simulink model "FCS_MPC_6ph_CIL_FCS_reduced"  (R2022a)
settings: Solver=ode23t  StartTime=0.0  StopTime=0.1  RelTol=1e-3  AbsTol=1e-3  EnableMultiTasking=on
values from neighbouring files (symbols this model uses):
  f_c = 100000    [Params_testbench.m]
  L_d = 0.0001473    [Params_testbench.m]
  L_q = 0.0001484    [Params_testbench.m]
  L_x = 0.00005566    (= 5.566e-05)    [Params_testbench.m]
  L_y = L_x    (= 5.566e-05)    [Params_testbench.m]
  p = 5    [Params_testbench.m]
  psi_pm = 0.0048    [Params_testbench.m]
  R_ph = 0.1278    [Params_testbench.m]
  u_dc = 36.0    (= 36)    [Params_testbench.m]
libraries: nesl_utility x39, fl_lib x32, hdlsllib x20, ee_lib x12, simulink x2, spsAlphaBetaZerotodq0Lib x1
(part 1 of 3)
settings Model: Creator=Michael Hoerner  LastModifiedBy=Andre Merx
settings SolverCC: AutoScaleAbsTol=off  AlgebraicLoopSolver=TrustRegion  DecoupledContinuousIntegration=on  MinimalZcImpactIntegration=on
settings DataIOCC: LimitDataPoints=on  MaxDataPoints=10000  ReturnWorkspaceOutputs=off
settings OptimizationCC: DefaultParameterBehavior=Inlined  PassReuseOutputArgsAs=Individual arguments  OptimizeBlockOrder=speed  DifferentSizesBufferReuse=on  EfficientTunableParamExpr=on
settings DebuggingCC: ParameterTunabilityLossMsg=error  UnconnectedInputMsg=warning  UnconnectedOutputMsg=warning  UnconnectedLineMsg=warning  AllowSymbolicDim=off  SFUnexpectedBacktrackingDiag=warning  SFNoUnconditionalDefaultTransitionDiag=warning  SFExecutionAtInitializationDiag=none  SFMachineParentedDataDiag=warning  ArithmeticOperatorsInVariantConditions=warning
settings HardwareCC: ProdBitPerPointer=32  ProdBitPerSizeT=32  ProdBitPerPtrDiffT=32  ProdLargestAtomicInteger=Long  ProdLargestAtomicFloat=Double  ProdWordSize=32  ProdHWDeviceType=ARM Compatible->ARM Cortex-R
settings SFSimCC: SimUseLocalCustomCode=off  MATLABDynamicMemAlloc=off  CustomCodeUndefinedFunction=UseInterfaceOnly
settings RTWCC: SystemTargetFile=ert.tlc  GenCodeOnly=on  TemplateMakefile=ert_default_tmf  GenerateReport=on  RTWUseLocalCustomCode=off  BuildConfiguration=Faster Runs  IncludeHyperlinkInReport=on  GenerateTraceInfo=on  GenerateTraceReport=on  GenerateTraceReportSl=on  GenerateTraceReportSf=on  GenerateTraceReportEml=on  GenerateCodeMetricsReport=on  CheckMdlBeforeBuild=Warning  DLArmComputeVersion=19.05
settings CodeAppCC: ForceParamTrailComments=on  IgnoreCustomStorageClasses=off  OperatorAnnotations=on  SimulinkDataObjDesc=on  SFDataObjDesc=on  MATLABFcnDesc=on  InsertBlockDesc=on  StateflowObjectComments=on  MATLABSourceComments=on  EnableCustomComments=on  ReqsInCode=on
settings ERTTargetCC: CodeReplacementLibrary=GNU C99 extensions  GenerateSampleERTMain=on  SuppressErrorStatus=on  IncludeFileDelimiter=UseQuote  CodeInterfacePackaging=Reusable function  SupportNonFinite=off  MultiInstanceErrorCode=Warning  RootIOFormat=Part of model data structure  ERTCustomFileTemplate=example_file_process.tlc  GlobalDataDefinition=InSourceFile  GlobalDataReference=InSourceFile  ERTFilePackagingFormat=CompactWithDataFile
settings ConfigComp: CovMetricSettings=dw  CovSaveCumulativeToWorkspaceVar=on  CovSaveSingleToWorkspaceVar=on  CovExternalEMLEnable=off  CovSFcnEnable=off
settings SimscapeCC: SimscapeLogDataHistory=10000

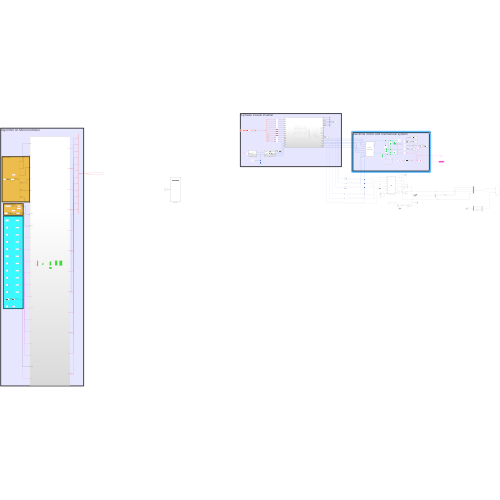
[thumbnail: Simulink's stored preview of the top-level diagram]
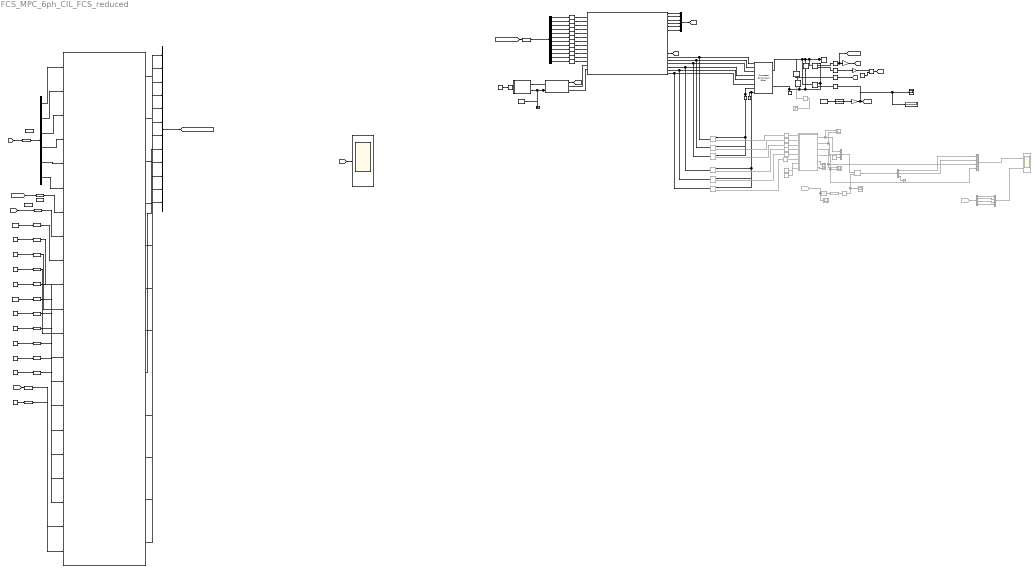
== system FCS_MPC_6ph_CIL_FCS_reduced ==
  note: electrical motor and mechanical system
  note: 6-phase 2-level inverter
  note: Von IP-Core ADC
  note: AXI
  note: Algorithm on Microcontroller
  note: Von IP-Core IncreEncoder
  6ph_Inverter : Subsystem
  6ph_PMSM_30deg_VSD1 : MATLAB Function  Commented=on  TreatAsAtomicUnit=on
  Alpha-Beta-Zero to dq0 : spsAlphaBetaZerotodq0Lib/Alpha-Beta-Zero to dq0  Commented=on  Alignment=Aligned with phase A axis
      settings: SourceProductBaseCode=PS
  Constant : Constant  Value=2*pi
  Constant10 : Constant  Commented=on  Value=1/3
  Constant11 : Constant  Value=R_ph
  Constant12 : Constant  Value=1/f_c
  Constant13 : Constant  Value=psi_pm
  Constant15 : Constant  Value=L_q
  Constant16 : Constant  Value=L_x
  Constant17 : Constant  Value=L_y
  Constant2 : Constant  Value=L_d
  Constant6 : Constant  Value=u_dc
  Constant8 : Constant  Commented=on  Value=0  OutDataTypeStr=single
  Constant9 : Constant  Commented=on
  DC_link : Subsystem
  Data Type Conversion{1..3,7,10..11,22..23,28..31,38..41} (16 alike) : DataTypeConversion  OutDataTypeStr=single  SaturateOnIntegerOverflow=off  RndMeth=Floor
  Data Type Conversion4 : DataTypeConversion  Commented=on  OutDataTypeStr=single  SaturateOnIntegerOverflow=off  RndMeth=Floor
  Data Type Conversion42 : DataTypeConversion  OutDataTypeStr=double  SaturateOnIntegerOverflow=off  RndMeth=Floor
  Data Type Conversion6 : DataTypeConversion  OutDataTypeStr=fixdt(1,24,11)  SaturateOnIntegerOverflow=off  RndMeth=Floor
  Data Type Conversion8 : DataTypeConversion  OutDataTypeStr=fixdt(1,24,20)  SaturateOnIntegerOverflow=off  RndMeth=Floor
  Data Type Conversion9 : DataTypeConversion  OutDataTypeStr=fixdt(1,18,11)  SaturateOnIntegerOverflow=off  RndMeth=Floor
  DelayValue1 : Delay  Commented=on  DelayLength=1
  Demux : Demux  Commented=on
  Demux1 : Demux  Commented=on  Outputs=3
  Demux2 : Demux  Outputs=12
  Demux6 : Demux  Outputs=6
  Display : Display
  Electrical Reference1 : fl_lib/Electrical/Electrical Elements/Electrical Reference
      settings: SourceProductBaseCode=PW,SS,VE
  From1 : From  Commented=on  GotoTag=theta_el
  From2 : From  Commented=on  GotoTag=v_opt
  Gain : Gain  Gain=30/pi
  Gain7 : Gain  Gain=p
  Gain8 : Gain  Gain=pi/30
  Ideal Angular Velocity Source1 : fl_lib/Mechanical/Mechanical Sources/Ideal Angular Velocity Source
      settings: SourceProductBaseCode=PW,SS,VE
  Ideal Rotational Motion Sensor1 : fl_lib/Mechanical/Mechanical Sensors/Ideal Rotational Motion Sensor  wrap_angle=simscape.enum.onoff.off  offset=0 deg
      settings: SourceProductBaseCode=PW,SS,VE
  Ideal Torque Sensor : fl_lib/Mechanical/Mechanical Sensors/Ideal Torque Sensor
      settings: SourceProductBaseCode=PW,SS,VE
  Ideal Torque Source : fl_lib/Mechanical/Mechanical Sources/Ideal Torque Source
      settings: SourceProductBaseCode=PW,SS,VE
  Inertia1 : fl_lib/Mechanical/Rotational Elements/Inertia  inertia=J kg*m^2  num_ports=foundation.enum.numPorts2.one  w_specify=off  w_priority=High  w=0 rad/s  w_nominal_specify=off  w_nominal_unit=rad/s  w_nominal_value=1  t_specify=off  t_priority=None  t=0 N*m  t_nominal_specify=off  t_nominal_unit=N*m  t_nominal_value=1
      settings: SourceProductBaseCode=PW,SS,VE
  Mechanical Rotational Reference1 : fl_lib/Mechanical/Rotational Elements/Mechanical Rotational Reference
      settings: SourceProductBaseCode=PW,SS,VE
  Microcontroller Software : Subsystem
  Mod : Math  Operator=mod
  Mux : Mux  Commented=on
  Mux1 : Mux  Inputs=6
  Mux2 : Mux  Commented=on
  Mux3 : Mux  Commented=on  Inputs=3
  Mux7 : Mux  Inputs=12
  Open Circuit : fl_lib/Electrical/Electrical Elements/Open Circuit  v_specify=off  v_priority=None  v=0 V  v_nominal_specify=off  v_nominal_unit=V  v_nominal_value=1
      settings: SourceProductBaseCode=PW,SS,VE
  Open Circuit1 : fl_lib/Electrical/Electrical Elements/Open Circuit  v_specify=off  v_priority=None  v=0 V  v_nominal_specify=off  v_nominal_unit=V  v_nominal_value=1
      settings: SourceProductBaseCode=PW,SS,VE
  PS-Simulink Converter{1..5,9} (6 alike) : nesl_utility/PS-Simulink Converter  Commented=on  PhysicalDomain=network_engine_domain  SubClassName=ps_output  LeftPortType=input  RightPortType=output  PseudoPeriodic=off  Frequencies=[]  VectorFormat=1-D array  Unit=V  AffineConversion=off
      settings: SourceProductBaseCode=SS,PW,VE
  PS-Simulink Converter6 : nesl_utility/PS-Simulink Converter  PhysicalDomain=network_engine_domain  SubClassName=ps_output  LeftPortType=input  RightPortType=output  PseudoPeriodic=off  Frequencies=[]  VectorFormat=1-D array  Unit=1  AffineConversion=off
      settings: SourceProductBaseCode=SS,PW,VE
  PS-Simulink Converter7 : nesl_utility/PS-Simulink Converter  PhysicalDomain=network_engine_domain  SubClassName=ps_output  LeftPortType=input  RightPortType=output  PseudoPeriodic=off  Frequencies=[]  VectorFormat=1-D array  Unit=1  AffineConversion=off
      settings: SourceProductBaseCode=SS,PW,VE
  PS-Simulink Converter8 : nesl_utility/PS-Simulink Converter  PhysicalDomain=network_engine_domain  SubClassName=ps_output  LeftPortType=input  RightPortType=output  PseudoPeriodic=off  Frequencies=[]  VectorFormat=1-D array  Unit=1  AffineConversion=off
      settings: SourceProductBaseCode=SS,PW,VE
  Power_Source : Subsystem
  Rotational Friction : fl_lib/Mechanical/Rotational Elements/Rotational Friction  brkwy_trq=0.0622476 N*m  brkwy_vel=0.1 rad/s  Col_trq=0.03460117 N*m  visc_coef=0.00026373 N*m/(rad/s)  w_specify=off  w_priority=None  w=0 rad/s  w_nominal_specify=off  w_nominal_unit=rad/s  w_nominal_value=1  t_specify=off  t_priority=None  t=0 N*m  t_nominal_specify=off  t_nominal_unit=N*m  t_nominal_value=1
      settings: SourceProductBaseCode=PW,SS,VE
  Scope : Scope
  Scope1 : Scope  Commented=on  NumInputPorts=2
  Scope2 : Scope  Commented=on  NumInputPorts=2
  Scope3 : Scope  Commented=on  NumInputPorts=2
  Scope4 : Scope  Commented=on
  Scope5 : Scope  Commented=on
  Simscape Component : SimscapeComponentBlock  SourceFile=SixPhase_PMSM  ComponentPath=SixPhase_PMSM  ComponentVariants=SixPhase_PMSM  ComponentVariantNames=SixPhase_PMSM  ClassName=SixPhase_PMSM  SchemaVersion=1  Rs=R_ph Ohm  Ld=L_d H  Lq=L_q H  Lx=L_x H  Ly=L_y H  psiPM=psi_pm Wb  np=p  theta_m_specify=off  theta_m_priority=None  theta_m=0 rad  theta_m_nominal_specify=off  theta_m_nominal_unit=rad  theta_m_nominal_value=1
      settings: CopyFcn=simscape.engine.sli.internal.componentblockcallback(gcbh,'COPY')  PreCopyFcn=simscape.engine.sli.internal.componentblockcallback(gcbh,'PRECOPY')  PreDeleteFcn=simscape.engine.sli.internal.componentblockcallback(gcbh,'PREDELETE')  InternalSimscapePortConfiguration="{\"Bottom\":[],\"Left\":[{\"id\":\"a1\",\"label\":\"a1\",\"type\":\"foundation.electrical.electrical\"},{\"id\":\"b1\",\"label\":\"b1\",\"type\":\"foundation.electrical.electrical\"},{\"id\":\"c1\",\"label\":\"c1\",\"type\":\"foundation.electrical.electrical\"},{\"id\":\"a2\",\"label\":\"a2\",\"type\":\"foundation.electrical.electrical\"},{\"id\":\"b2\",\"label\":\"b2\",\"type\":\"foundation.electrical.electrical\"},{\"id\":\"c2\",\"label\":\"c2\",\"type\":\"foundation.electrical.electrical\"},{\"id\":\"n1\",\"label\":\"n1\",\"type\":\"foundation.electrical.electrical\"},{\"id\":\"n2\",\"label\":\"n2\",\"type\":\"foundation.electrical.electrical\"}],\"Right\":[{\"id\":\"R\",\"label\":\"R\",\"type\":\"foundation.mechanical.rotational.rotational\"},{\"id\":\"C\",\"label\":\"C\",\"type\":\"foundation.mechanical.rotational.rotational\"}],\"Top\":[]}"
      mask Type: SixPhase_PMSM
  Simulink-PS Converter{,2..7,11..12,17..20} (13 alike) : nesl_utility/Simulink-PS Converter  PhysicalDomain=network_engine_domain  SubClassName=ps_input  LeftPortType=input  RightPortType=output  PseudoPeriodic=off  Frequencies=[]  NoiseDistribution=none  NoiseParameters=[]  Unit=1  AffineConversion=off  FilteringAndDerivatives=provide  SimscapeFilterOrder=1  InputFilterTimeConstant=0.001  UdotUserProvided=0
      settings: SourceProductBaseCode=SS,PW,VE
  Simulink-PS Converter1 : nesl_utility/Simulink-PS Converter  Commented=on  PhysicalDomain=network_engine_domain  SubClassName=ps_input  LeftPortType=input  RightPortType=output  PseudoPeriodic=off  Frequencies=[]  NoiseDistribution=none  NoiseParameters=[]  Unit=1  AffineConversion=off  FilteringAndDerivatives=filter  SimscapeFilterOrder=1  InputFilterTimeConstant=0.001  UdotUserProvided=0
      settings: SourceProductBaseCode=SS,PW,VE
  Simulink-PS Converter10 : nesl_utility/Simulink-PS Converter  PhysicalDomain=network_engine_domain  SubClassName=ps_input  LeftPortType=input  RightPortType=output  PseudoPeriodic=off  Frequencies=[]  NoiseDistribution=none  NoiseParameters=[]  Unit=1  AffineConversion=off  FilteringAndDerivatives=filter  SimscapeFilterOrder=1  InputFilterTimeConstant=0.001  UdotUserProvided=0
      settings: SourceProductBaseCode=SS,PW,VE
  Solver Configuration1 : nesl_utility/Solver Configuration  PhysicalDomain=network_engine_domain  SubClassName=solver  LeftPortType=input  RightPortType=generic  Tones=[]  Harmonics=[]  SimulateNoise=off  Profile=off  UseLocalSampling=off  EnableSwitchedLinearOptims=on  FrequencyDomain=off  UseCCode=off  RelTol=0.001  AbsTol=1e-06  MinStep=1e-09  ToWorkspace=off  RevertToSquareIcSolve=off  NumHomotopyIterations=100  PhasorMode=off  PhasorModeNumHarmonics=1  IndexReductionMethod=DerivativeReplacement  DoDC=off  ResidualTolerance=1e-09  UseLocalSolver=off  LocalSolverChoice=NE_BACKWARD_EULER_ADVANCER  LocalSolverSampleTime=1e-6  DoFixedCost=off  MaxNonlinIter=3  MaxModeIter=2  ComputeImpulses=off  ImpulseIterations=2  LinearAlgebra=Sparse  LinearAlgebraNumThread=0  EquationFormulation=NE_TIME_EF  DelaysMemoryBudget=1024  AutomaticFiltering=on  FilteringTimeConstant=0.001  PartitionStorageMethod=AS_NEEDED  PartitionMemoryBudget=1024  PartitionMethod=FAST
      settings: SourceProductBaseCode=SS,PW,VE
  Step1 : Step  Commented=on  Time=0.08  After=-0.5  SampleTime=0
  Terminator5 : Terminator  Commented=on
  Terminator6 : Terminator  Commented=on
  Terminator7 : Terminator  Commented=on
  Transfer Fcn : TransferFcn  Denominator=[0.0005 1]
  Unit Delay1 : UnitDelay  Commented=on  SampleTime=1/f_c  HasFrameUpgradeWarning=on
  Voltage Sensor{,1..5} (6 alike) : fl_lib/Electrical/Electrical Sensors/Voltage Sensor  Commented=on
      settings: SourceProductBaseCode=PW,SS,VE
  id_ref1 : Constant  Value=0
  iq_ref1 : Constant  Value=10
  ix_ref : Constant  Value=0
  iy_ref : Constant  Value=0
  n_ref : Constant  Value=3000
  phase_currents : Scope
  pole_pairs : Constant  Value=p
  wires:
  DC_link/1(u_dc_link_measured) -> [u_dc_link]
  Constant6/1 -> Simulink-PS Converter/1
  PS-Simulink Converter7/1 -> Gain7/1  "theta_m"
  Gain7/1 -> Mod/1  "theta_el"
  Gain8/1 -> Simulink-PS Converter10/1, Display/1, Scope/1, [omega_m]
  PS-Simulink Converter6/1 -> Gain/1, [omega_m_m]  "omega_m"
  PS-Simulink Converter8/1 -> [torque]
  [i_ph] -> phase_currents/1
  n_ref/1 -> Transfer Fcn/1
  Gain/1 -> [n_RPM]
  Step1/1 -> Simulink-PS Converter1/1
  6ph_Inverter/1(i_1) -> Mux1/1  "i_a1"
  6ph_Inverter/6(i_6) -> Mux1/6  "i_c2"
  6ph_Inverter/4(i_4) -> Mux1/4  "i_a2"
  Demux2/6 -> Simulink-PS Converter17/1
  Demux2/5 -> Simulink-PS Converter7/1
  6ph_Inverter/13(i_dc) -> [i_dc]
  Demux2/7 -> Simulink-PS Converter18/1
  6ph_Inverter/3(i_3) -> Mux1/3  "i_c1"
  6ph_Inverter/5(i_5) -> Mux1/5  "i_b2"
  Demux2/3 -> Simulink-PS Converter5/1
  [Switching_states_IP_Cores] -> Data Type Conversion42/1
  6ph_Inverter/2(i_2) -> Mux1/2  "i_b1"
  Demux2/2 -> Simulink-PS Converter4/1
  Demux2/11 -> Simulink-PS Converter11/1
  Demux2/12 -> Simulink-PS Converter12/1
  Demux2/8 -> Simulink-PS Converter19/1
  Demux2/9 -> Simulink-PS Converter20/1
  Demux2/4 -> Simulink-PS Converter6/1
  Demux2/10 -> Simulink-PS Converter3/1
  Demux2/1 -> Simulink-PS Converter2/1
  Mux1/1 -> [i_ph]
  Constant/1 -> Mod/2
  Mod/1 -> [theta_el]
  iq_ref1/1 -> Data Type Conversion30/1
  Data Type Conversion30/1 -> Microcontroller Software/17(iq_ref)
  Constant11/1 -> Data Type Conversion22/1
  Constant13/1 -> Data Type Conversion28/1
  [u_dc_link] -> Data Type Conversion7/1
  Data Type Conversion10/1 -> Microcontroller Software/10(Ld)
  Demux6/1 -> Microcontroller Software/1(i_a1)
  Data Type Conversion23/1 -> Microcontroller Software/15(SampleTime)
  Data Type Conversion22/1 -> Microcontroller Software/9(Rs)
  Constant12/1 -> Data Type Conversion23/1
  id_ref1/1 -> Data Type Conversion29/1
  Constant2/1 -> Data Type Conversion10/1
  Data Type Conversion29/1 -> Microcontroller Software/16(id_ref)
  Demux6/2 -> Microcontroller Software/2(i_b1)
  Demux6/3 -> Microcontroller Software/3(i_c1)
  Data Type Conversion28/1 -> Microcontroller Software/14(psiPM)
  Constant15/1 -> Data Type Conversion11/1
  Data Type Conversion11/1 -> Microcontroller Software/11(Lq)
  Demux6/4 -> Microcontroller Software/4(i_a2)
  Demux6/5 -> Microcontroller Software/5(i_b2)
  Demux6/6 -> Microcontroller Software/6(i_c2)
  Constant16/1 -> Data Type Conversion31/1
  Data Type Conversion31/1 -> Microcontroller Software/12(Lx)
  Constant17/1 -> Data Type Conversion38/1
  Data Type Conversion38/1 -> Microcontroller Software/13(Ly)
  pole_pairs/1 -> Data Type Conversion41/1
  Data Type Conversion39/1 -> Microcontroller Software/18(ix_ref)
  ix_ref/1 -> Data Type Conversion39/1
  Data Type Conversion40/1 -> Microcontroller Software/19(iy_ref)
  iy_ref/1 -> Data Type Conversion40/1
  Data Type Conversion41/1 -> Microcontroller Software/21(pole_pairs)
  Microcontroller Software/1(HB1T1) -> Mux7/1
  Microcontroller Software/2(HB1B1) -> Mux7/2
  Microcontroller Software/3(HB2T1) -> Mux7/3
  Microcontroller Software/4(HB2B1) -> Mux7/4
  Microcontroller Software/5(HB3T1) -> Mux7/5
  Microcontroller Software/6(HB3B1) -> Mux7/6
  Microcontroller Software/7(HB4T) -> Mux7/7
  Microcontroller Software/8(HB4B) -> Mux7/8
  Microcontroller Software/9(HB5T) -> Mux7/9
  Microcontroller Software/10(HB5B) -> Mux7/10
  Microcontroller Software/11(HB6T) -> Mux7/11
  Microcontroller Software/12(HB6B) -> Mux7/12
  Mux7/1 -> [Switching_states_IP_Cores]
  Data Type Conversion42/1 -> Demux2/1
  Constant9/1 -> 6ph_PMSM_30deg_VSD1/8(c6)
  6ph_PMSM_30deg_VSD1/6(y6) -> Terminator6/1
  6ph_PMSM_30deg_VSD1/3(y3) -> Mux/3, Scope2/1  "v_x_inverter"
  Constant10/1 -> 6ph_PMSM_30deg_VSD1/7(k6)
  6ph_PMSM_30deg_VSD1/1(y1) -> Scope3/1, Mux3/1  "i_alpha"
  6ph_PMSM_30deg_VSD1/2(y2) -> Scope3/2, Mux3/2  "i_beta"
  6ph_PMSM_30deg_VSD1/4(y4) -> Scope2/2, Mux/4  "v_y_inverter"
  Mux3/1 -> Alpha-Beta-Zero to dq0/1
  Constant8/1 -> Mux3/3
  6ph_PMSM_30deg_VSD1/5(y5) -> Terminator5/1
  Demux1/2 -> Mux/2  "v_q_inverter"
  Demux1/3 -> Terminator7/1
  Alpha-Beta-Zero to dq0/1 -> Demux1/1
  Demux1/1 -> Mux/1  "v_d_inverter"
  PS-Simulink Converter1/1 -> 6ph_PMSM_30deg_VSD1/1(u1)
  PS-Simulink Converter2/1 -> 6ph_PMSM_30deg_VSD1/2(u2)
  PS-Simulink Converter3/1 -> 6ph_PMSM_30deg_VSD1/3(u3)
  PS-Simulink Converter4/1 -> 6ph_PMSM_30deg_VSD1/4(u4)
  PS-Simulink Converter5/1 -> 6ph_PMSM_30deg_VSD1/5(u5)
  PS-Simulink Converter9/1 -> 6ph_PMSM_30deg_VSD1/6(u6)
  Unit Delay1/1 -> Data Type Conversion4/1
  Data Type Conversion4/1 -> DelayValue1/1
  Mux/1 -> Scope1/1
  From2/1 -> Demux/1
  Demux/1 -> Mux2/1  "v_d_MPC"
  Demux/2 -> Mux2/2  "v_q_MPC"
  Demux/3 -> Mux2/3  "v_x_MPC"
  Demux/4 -> Mux2/4  "v_y_MPC"
  Mux2/1 -> Scope1/2
  From1/1 -> Scope5/1, Unit Delay1/1  "End_Cycle"
  DelayValue1/1 -> Alpha-Beta-Zero to dq0/2, Scope4/1  "End_Cycle"
  [i_ph] -> Data Type Conversion1/1  "End_Cycle"
  [theta_el] -> Data Type Conversion3/1  "End_Cycle"
  [omega_m_m] -> Data Type Conversion2/1  "fc"
  Data Type Conversion7/1 -> Microcontroller Software/20(u_dc_link)
  Data Type Conversion1/1 -> Demux6/1  "fc"
  Data Type Conversion3/1 -> Microcontroller Software/8(theta_el)
  Data Type Conversion2/1 -> Microcontroller Software/7(omega_m)
  Transfer Fcn/1 -> Gain8/1
  connections:
  DC_link/LConn2 -- Power_Source/RConn2 -- Solver Configuration1/RConn1 -- Electrical Reference1/LConn1
  Inertia1/LConn1 -- Ideal Torque Sensor/LConn1 -- Simscape Component/RConn1 -- Ideal Angular Velocity Source1/LConn1 -- Rotational Friction/LConn1 -- Ideal Rotational Motion Sensor1/LConn1
  Ideal Rotational Motion Sensor1/RConn1 -- Ideal Angular Velocity Source1/RConn2 -- Rotational Friction/RConn1 -- Simscape Component/RConn2 -- Mechanical Rotational Reference1/LConn1 -- Ideal Torque Source/RConn2
  Power_Source/RConn1 -- DC_link/LConn1
  PS-Simulink Converter6/LConn1 -- Ideal Rotational Motion Sensor1/RConn2
  Simulink-PS Converter/RConn1 -- Power_Source/LConn1
  6ph_Inverter/LConn13 -- DC_link/RConn1
  6ph_Inverter/LConn14 -- DC_link/RConn2
  PS-Simulink Converter7/LConn1 -- Ideal Rotational Motion Sensor1/RConn3
  Simulink-PS Converter10/RConn1 -- Ideal Angular Velocity Source1/RConn1
  PS-Simulink Converter8/LConn1 -- Ideal Torque Sensor/RConn2
  Simulink-PS Converter1/RConn1 -- Ideal Torque Source/RConn1
  Ideal Torque Source/LConn1 -- Ideal Torque Sensor/RConn1
  Simscape Component/LConn8 -- Voltage Sensor5/RConn2 -- Voltage Sensor4/RConn2 -- Voltage Sensor3/RConn2 -- Open Circuit1/LConn1
  6ph_Inverter/RConn2 -- Voltage Sensor1/LConn1 -- Simscape Component/LConn2
  Simscape Component/LConn7 -- Voltage Sensor2/RConn2 -- Voltage Sensor1/RConn2 -- Voltage Sensor/RConn2 -- Open Circuit/LConn1
  6ph_Inverter/RConn1 -- Simscape Component/LConn1 -- Voltage Sensor/LConn1
  6ph_Inverter/RConn4 -- Voltage Sensor3/LConn1 -- Simscape Component/LConn4
  6ph_Inverter/RConn5 -- Voltage Sensor4/LConn1 -- Simscape Component/LConn5
  Simulink-PS Converter7/RConn1 -- 6ph_Inverter/LConn5
  Simulink-PS Converter12/RConn1 -- 6ph_Inverter/LConn12
  Simulink-PS Converter20/RConn1 -- 6ph_Inverter/LConn9
  Simulink-PS Converter17/RConn1 -- 6ph_Inverter/LConn6
  Simulink-PS Converter11/RConn1 -- 6ph_Inverter/LConn11
  Simulink-PS Converter19/RConn1 -- 6ph_Inverter/LConn8
  Simulink-PS Converter6/RConn1 -- 6ph_Inverter/LConn4
  Simulink-PS Converter3/RConn1 -- 6ph_Inverter/LConn10
  Simulink-PS Converter4/RConn1 -- 6ph_Inverter/LConn2
  Simscape Component/LConn3 -- 6ph_Inverter/RConn3 -- Voltage Sensor2/LConn1
  Simscape Component/LConn6 -- Voltage Sensor5/LConn1 -- 6ph_Inverter/RConn6
  Simulink-PS Converter5/RConn1 -- 6ph_Inverter/LConn3
  Simulink-PS Converter2/RConn1 -- 6ph_Inverter/LConn1
  Simulink-PS Converter18/RConn1 -- 6ph_Inverter/LConn7
  Voltage Sensor/RConn1 -- PS-Simulink Converter1/LConn1
  Voltage Sensor1/RConn1 -- PS-Simulink Converter2/LConn1
  Voltage Sensor2/RConn1 -- PS-Simulink Converter3/LConn1
  Voltage Sensor3/RConn1 -- PS-Simulink Converter4/LConn1
  Voltage Sensor4/RConn1 -- PS-Simulink Converter5/LConn1
  Voltage Sensor5/RConn1 -- PS-Simulink Converter9/LConn1

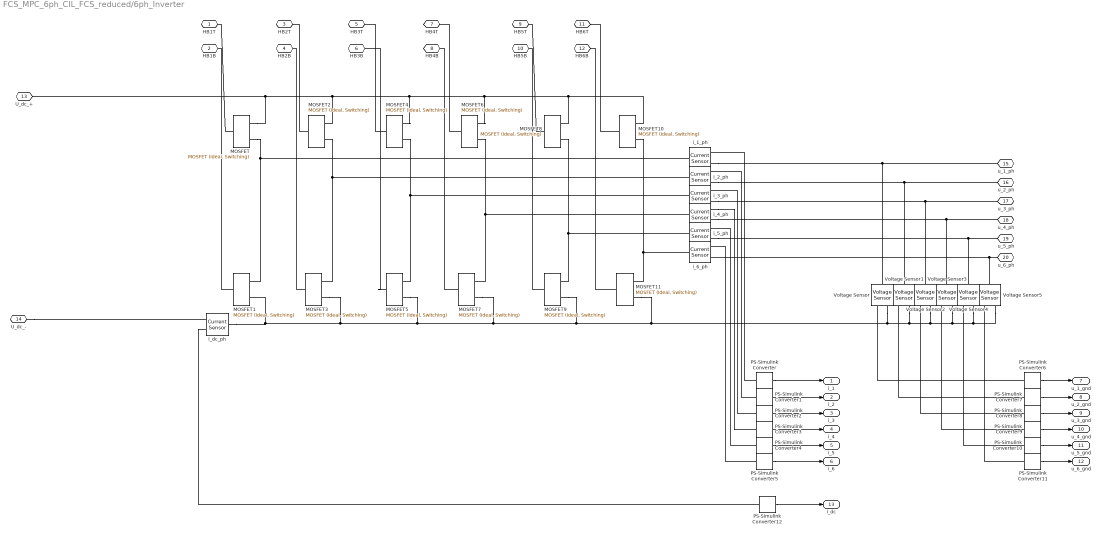
== system FCS_MPC_6ph_CIL_FCS_reduced/6ph_Inverter ==
  MOSFET{,1..11} (12 alike) : ee_lib/Semiconductors & Converters/MOSFET (Ideal, Switching)  Rds=RDSon Ohm  Goff=1e-6 1/Ohm  Vth=0.7 V  diode_param=1  diode_Vf=0.8 V  diode_Ron=0.001 Ohm  diode_Goff=1e-5 1/Ohm  diode_C=5e-8 F  diode_iRM=-235 A  diode_iF=300 A  diode_idot=-50 A/us  diode_trr_param=1  diode_trr_factor=3  diode_trr=15 us  diode_Qrr=1.5e+3 s*uA  thermal_loss_option=ee.enum.converters.thermalLossOption.constantvalues  Von_data=[0, 1.1, 1.3, 1.45, 1.75, 2.25, 2.7; 0, 1, 1.15, 1.35, 1.7, 2.35, 3] V  Tj=[298.15, 398.15] K  Iout_data=[0, 10, 50, 100, 200, 400, 600] A  Eon_data=[0, .29, 1.43, 2.86, 5.71, 13.14, 22.86; 0, .57, 2.63, 5.14, 10.29, 20.57, 30.29] * 1e-3 J  Eoff_data=[0, .21, 1.07, 2.14, 4.29, 9.86, 17.14; 0, .43, 1.97, 3.86, 7.71, 15.43, 22.71] * 1e-3 J  Tj_loss=[298.15, 398.15] K  Iout_data_loss=[0, 10, 50, 100, 200, 400, 600] A  Eon_scalar=22.86e-3 J  Eoff_scalar=17.14e-3 J  Voff=300 V  Iout_scalar=600 A  diodeModelType=ee.enum.converters.diodeModelType.pwl  diodeTableType=ee.enum.diode.tableType.IfMat  diode_IfMat=[.07, .12, .19, 1.75, 4.24, 7.32, 11.2; .16, .3, .72, 2.14, 4.02, 6.35, 9.12] A  diode_VfMat=[.9, 1.15, 1.25, 1.5, 1.75, 2.17, 2.6, 2.85; .58, .68, .75, 1.1, 1.38, 1.77, 2.27, 2.7] V  diode_TjVec=[25, 125] degC  diode_VfVec=[.5, .7, .9, 1.3, 1.7, 2.1, 2.5] V  diode_IfVec=[.1, .2, .5, 1, 2, 4, 7, 10] A  diode_Vr=-600 V  diode_Ls=150 nH  diode_Erec=0.03 J  thermal_network_parameterization=ee.enum.thermalNetworkTopology.external  Rth=[.03, .2] K/W  Rth_Cauer=[.03, .1, .2] K/W  Rth_Foster=[.03, .2] K/W  thermal_mass_parameterization=ee.enum.thermalNetwork.timeconstant  thermal_mass=[3, 25] J/K  thermal_mass_Cauer=[3, 10, 25] J/K  thermal_mass_Foster=[33, 50] J/K  thermal_time_constant=[.1, 5] s  thermal_time_constant_Cauer=[.1, 1, 5] s  thermal_time_constant_Foster=[1, 10] s  thermal_mass_initial_temperatures=[25, 25] degC  thermal_mass_initial_temperatures_Cauer=[25, 25, 25] degC  junction_thermal_mass=0.1 J/K  steadyState_Foster=simscape.enum.onoff.on  Tvec_initial_Foster=[25, 25, 25, 25] degC  no_thermal_network=0  junction_temperature_specify=off  junction_temperature_priority=None  junction_temperature=25 degC  junction_temperature_nominal_specify=off  junction_temperature_nominal_unit=degC  junction_temperature_nominal_value=1  vT_specify=off  vT_priority=None  vT=0 V  vT_nominal_specify=off  vT_nominal_unit=V  vT_nominal_value=1  Qj_specify=off  Qj_priority=None  Qj=0 W  Qj_nominal_specify=off  Qj_nominal_unit=W  Qj_nominal_value=1
  PS-Simulink Converter{,1..5,12} (7 alike) : nesl_utility/PS-Simulink Converter  PhysicalDomain=network_engine_domain  SubClassName=ps_output  LeftPortType=input  RightPortType=output  PseudoPeriodic=off  Frequencies=[]  VectorFormat=1-D array  Unit=A  AffineConversion=off
      settings: SourceProductBaseCode=SS,PW,VE
  PS-Simulink Converter{6..11} (6 alike) : nesl_utility/PS-Simulink Converter  PhysicalDomain=network_engine_domain  SubClassName=ps_output  LeftPortType=input  RightPortType=output  PseudoPeriodic=off  Frequencies=[]  VectorFormat=1-D array  Unit=V  AffineConversion=off
      settings: SourceProductBaseCode=SS,PW,VE
  Voltage Sensor{,1..5} (6 alike) : fl_lib/Electrical/Electrical Sensors/Voltage Sensor
      settings: SourceProductBaseCode=PW,SS,VE
  i_1_ph : fl_lib/Electrical/Electrical Sensors/Current Sensor
      settings: SourceProductBaseCode=PW,SS,VE
  i_2_ph : fl_lib/Electrical/Electrical Sensors/Current Sensor
      settings: SourceProductBaseCode=PW,SS,VE
  i_3_ph : fl_lib/Electrical/Electrical Sensors/Current Sensor
      settings: SourceProductBaseCode=PW,SS,VE
  i_4_ph : fl_lib/Electrical/Electrical Sensors/Current Sensor
      settings: SourceProductBaseCode=PW,SS,VE
  i_5_ph : fl_lib/Electrical/Electrical Sensors/Current Sensor
      settings: SourceProductBaseCode=PW,SS,VE
  i_6_ph : fl_lib/Electrical/Electrical Sensors/Current Sensor
      settings: SourceProductBaseCode=PW,SS,VE
  i_dc_ph : fl_lib/Electrical/Electrical Sensors/Current Sensor
      settings: SourceProductBaseCode=PW,SS,VE
  HB1T : PMIOPort  Side=Left
  HB1B : PMIOPort  Port=2  Side=Left
  HB2T : PMIOPort  Port=3  Side=Left
  HB2B : PMIOPort  Port=4  Side=Left
  HB3T : PMIOPort  Port=5  Side=Left
  HB3B : PMIOPort  Port=6  Side=Left
  HB4T : PMIOPort  Port=7  Side=Left
  HB4B : PMIOPort  Port=8  Side=Left
  HB5T : PMIOPort  Port=9  Side=Left
  HB5B : PMIOPort  Port=10  Side=Left
  HB6T : PMIOPort  Port=11  Side=Left
  HB6B : PMIOPort  Port=12  Side=Left
  U_dc_+ : PMIOPort  Port=13  Side=Left
  U_dc_- : PMIOPort  Port=14  Side=Left
  u_1_ph : PMIOPort  Port=15  Side=Right
  u_2_ph : PMIOPort  Port=16  Side=Right
  u_3_ph : PMIOPort  Port=17  Side=Right
  u_4_ph : PMIOPort  Port=18  Side=Right
  u_5_ph : PMIOPort  Port=19  Side=Right
  u_6_ph : PMIOPort  Port=20  Side=Right
  i_1 : Outport  VectorParamsAs1DForOutWhenUnconnected=off
  i_2 : Outport  Port=2  VectorParamsAs1DForOutWhenUnconnected=off
  i_3 : Outport  Port=3  VectorParamsAs1DForOutWhenUnconnected=off
  i_4 : Outport  Port=4  VectorParamsAs1DForOutWhenUnconnected=off
  i_5 : Outport  Port=5  VectorParamsAs1DForOutWhenUnconnected=off
  i_6 : Outport  Port=6  VectorParamsAs1DForOutWhenUnconnected=off
  u_1_gnd : Outport  Port=7  VectorParamsAs1DForOutWhenUnconnected=off
  u_2_gnd : Outport  Port=8  VectorParamsAs1DForOutWhenUnconnected=off
  u_3_gnd : Outport  Port=9  VectorParamsAs1DForOutWhenUnconnected=off
  u_4_gnd : Outport  Port=10  VectorParamsAs1DForOutWhenUnconnected=off
  u_5_gnd : Outport  Port=11  VectorParamsAs1DForOutWhenUnconnected=off
  u_6_gnd : Outport  Port=12  VectorParamsAs1DForOutWhenUnconnected=off
  i_dc : Outport  Port=13  VectorParamsAs1DForOutWhenUnconnected=off
  wires:
  PS-Simulink Converter/1 -> i_1/1
  PS-Simulink Converter1/1 -> i_2/1
  PS-Simulink Converter2/1 -> i_3/1
  PS-Simulink Converter3/1 -> i_4/1
  PS-Simulink Converter4/1 -> i_5/1
  PS-Simulink Converter5/1 -> i_6/1
  PS-Simulink Converter9/1 -> u_4_gnd/1
  PS-Simulink Converter8/1 -> u_3_gnd/1
  PS-Simulink Converter7/1 -> u_2_gnd/1
  PS-Simulink Converter6/1 -> u_1_gnd/1
  PS-Simulink Converter10/1 -> u_5_gnd/1
  PS-Simulink Converter11/1 -> u_6_gnd/1
  PS-Simulink Converter12/1 -> i_dc/1
  connections:
  MOSFET6/RConn2 -- i_4_ph/LConn1 -- MOSFET7/RConn1
  MOSFET2/RConn2 -- i_2_ph/LConn1 -- MOSFET3/RConn1
  MOSFET4/RConn2 -- i_3_ph/LConn1 -- MOSFET5/RConn1
  MOSFET5/RConn2 -- Voltage Sensor5/RConn2 -- Voltage Sensor4/RConn2 -- Voltage Sensor3/RConn2 -- Voltage Sensor2/RConn2 -- Voltage Sensor1/RConn2 -- Voltage Sensor/RConn2 -- MOSFET11/RConn2 -- MOSFET9/RConn2 -- MOSFET7/RConn2 -- i_dc_ph/LConn1 -- MOSFET1/RConn2 -- MOSFET3/RConn2
  MOSFET/RConn2 -- i_1_ph/LConn1 -- MOSFET1/RConn1
  MOSFET11/LConn1 -- HB6B/RConn1
  MOSFET8/RConn2 -- i_5_ph/LConn1 -- MOSFET9/RConn1
  MOSFET2/LConn1 -- HB2T/RConn1
  MOSFET10/RConn2 -- i_6_ph/LConn1 -- MOSFET11/RConn1
  MOSFET/LConn1 -- HB1T/RConn1
  MOSFET9/LConn1 -- HB5B/RConn1
  MOSFET5/LConn1 -- HB3B/RConn1
  MOSFET1/LConn1 -- HB1B/RConn1
  MOSFET7/LConn1 -- HB4B/RConn1
  MOSFET8/LConn1 -- HB5T/RConn1
  MOSFET4/LConn1 -- HB3T/RConn1
  MOSFET10/LConn1 -- HB6T/RConn1
  MOSFET6/LConn1 -- HB4T/RConn1
  MOSFET3/LConn1 -- HB2B/RConn1
  i_1_ph/RConn2 -- Voltage Sensor/LConn1 -- u_1_ph/RConn1
  i_2_ph/RConn2 -- u_2_ph/RConn1 -- Voltage Sensor1/LConn1
  i_3_ph/RConn2 -- u_3_ph/RConn1 -- Voltage Sensor2/LConn1
  i_4_ph/RConn2 -- Voltage Sensor3/LConn1 -- u_4_ph/RConn1
  i_5_ph/RConn2 -- Voltage Sensor4/LConn1 -- u_5_ph/RConn1
  u_6_ph/RConn1 -- i_6_ph/RConn2 -- Voltage Sensor5/LConn1
  PS-Simulink Converter/LConn1 -- i_1_ph/RConn1
  PS-Simulink Converter1/LConn1 -- i_2_ph/RConn1
  PS-Simulink Converter2/LConn1 -- i_3_ph/RConn1
  i_4_ph/RConn1 -- PS-Simulink Converter3/LConn1
  PS-Simulink Converter4/LConn1 -- i_5_ph/RConn1
  PS-Simulink Converter5/LConn1 -- i_6_ph/RConn1
  PS-Simulink Converter6/LConn1 -- Voltage Sensor/RConn1
  PS-Simulink Converter7/LConn1 -- Voltage Sensor1/RConn1
  PS-Simulink Converter8/LConn1 -- Voltage Sensor2/RConn1
  PS-Simulink Converter9/LConn1 -- Voltage Sensor3/RConn1
  PS-Simulink Converter10/LConn1 -- Voltage Sensor4/RConn1
  PS-Simulink Converter11/LConn1 -- Voltage Sensor5/RConn1
  U_dc_-/RConn1 -- i_dc_ph/RConn2
  PS-Simulink Converter12/LConn1 -- i_dc_ph/RConn1
  MOSFET6/RConn1 -- MOSFET/RConn1 -- U_dc_+/RConn1 -- MOSFET2/RConn1 -- MOSFET4/RConn1 -- MOSFET10/RConn1 -- MOSFET8/RConn1

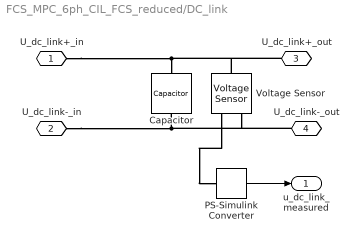
== system FCS_MPC_6ph_CIL_FCS_reduced/DC_link ==
  Capacitor : fl_lib/Electrical/Electrical Elements/Capacitor  c=C_dc_link uF  r=1e-6 Ohm  g=0 1/Ohm  i_specify=off  i_priority=None  i=0 A  i_nominal_specify=off  i_nominal_unit=A  i_nominal_value=1  v_specify=off  v_priority=None  v=0 V  v_nominal_specify=off  v_nominal_unit=V  v_nominal_value=1  vc_specify=off  vc_priority=High  vc=0 V  vc_nominal_specify=off  vc_nominal_unit=V  vc_nominal_value=1
      settings: SourceProductBaseCode=PW,SS,VE
  PS-Simulink Converter : nesl_utility/PS-Simulink Converter  PhysicalDomain=network_engine_domain  SubClassName=ps_output  LeftPortType=input  RightPortType=output  PseudoPeriodic=off  Frequencies=[]  VectorFormat=1-D array  Unit=1  AffineConversion=off
      settings: SourceProductBaseCode=SS,PW,VE
  Voltage Sensor : fl_lib/Electrical/Electrical Sensors/Voltage Sensor
      settings: SourceProductBaseCode=PW,SS,VE
  U_dc_link+_in : PMIOPort  Side=Left
  U_dc_link-_in : PMIOPort  Port=2  Side=Left
  U_dc_link+_out : PMIOPort  Port=3  Side=Right
  U_dc_link-_out : PMIOPort  Port=4  Side=Right
  u_dc_link_measured : Outport  VectorParamsAs1DForOutWhenUnconnected=off
  wires:
  PS-Simulink Converter/1 -> u_dc_link_measured/1
  connections:
  U_dc_link+_in/RConn1 -- Voltage Sensor/LConn1 -- U_dc_link+_out/RConn1 -- Capacitor/LConn1
  U_dc_link-_in/RConn1 -- Voltage Sensor/RConn2 -- U_dc_link-_out/RConn1 -- Capacitor/RConn1
  Voltage Sensor/RConn1 -- PS-Simulink Converter/LConn1

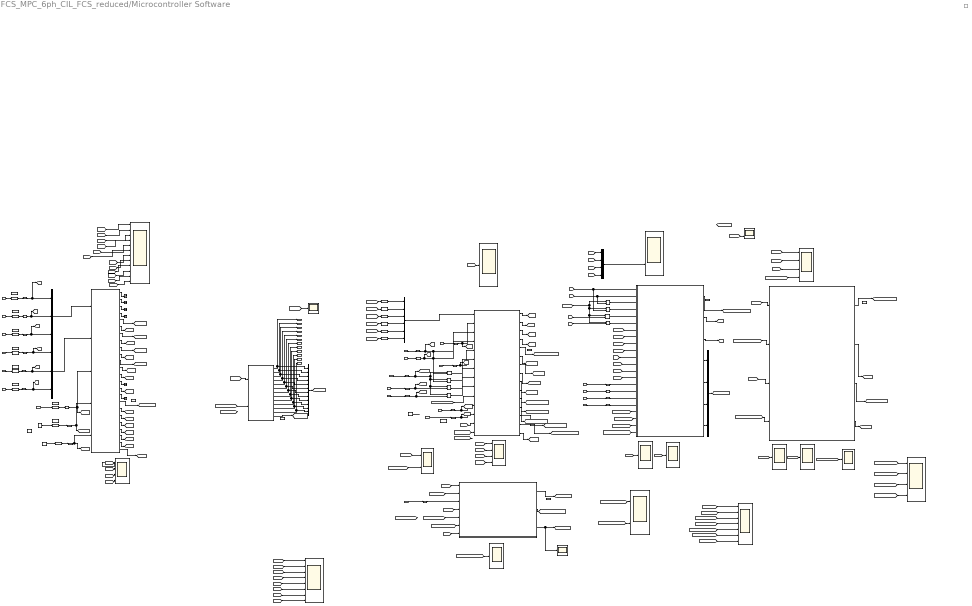
== system FCS_MPC_6ph_CIL_FCS_reduced/Microcontroller Software ==
  i_a1 : Inport
  i_b1 : Inport  Port=2
  i_c1 : Inport  Port=3
  i_a2 : Inport  Port=4
  i_b2 : Inport  Port=5
  i_c2 : Inport  Port=6
  omega_m : Inport  Port=7
  theta_el : Inport  Port=8
  Rs : Inport  Port=9
  Ld : Inport  Port=10
  Lq : Inport  Port=11
  Lx : Inport  Port=12
  Ly : Inport  Port=13
  psiPM : Inport  Port=14
  SampleTime : Inport  Port=15
  id_ref : Inport  Port=16
  iq_ref : Inport  Port=17
  ix_ref : Inport  Port=18
  iy_ref : Inport  Port=19
  u_dc_link : Inport  Port=20
  pole_pairs : Inport  Port=21
  Ablauf : Scope  NumInputPorts=7
  Constant : Constant  Value=314  OutDataTypeStr=single  SampleTime=-1
  Constant1 : Constant  Value=0  OutDataTypeStr=single  SampleTime=1/100000000
  Constant2 : Constant  Value=0  OutDataTypeStr=fixdt(1,24,20)  SampleTime=-1
  Data Type Conversion1 : DataTypeConversion  OutDataTypeStr=fixdt(1,24,11)  SaturateOnIntegerOverflow=off  RndMeth=Floor
  Data Type Conversion10 : DataTypeConversion  OutDataTypeStr=fixdt(1,18,14)  SaturateOnIntegerOverflow=off  RndMeth=Floor
  Data Type Conversion11 : DataTypeConversion  OutDataTypeStr=fixdt(1,18,14)  SaturateOnIntegerOverflow=off  RndMeth=Floor
  Data Type Conversion12 : DataTypeConversion  OutDataTypeStr=fixdt(1,24,20)  SaturateOnIntegerOverflow=off  RndMeth=Floor
  Data Type Conversion{13..18} (6 alike) : DataTypeConversion  OutDataTypeStr=fixdt(1,18,11)  SaturateOnIntegerOverflow=off  RndMeth=Floor
  Data Type Conversion{2..3,5..7,9,19..24} (12 alike) : DataTypeConversion  OutDataTypeStr=fixdt(1,27,18)  SaturateOnIntegerOverflow=off  RndMeth=Floor
  Data Type Conversion4 : DataTypeConversion  OutDataTypeStr=boolean  RndMeth=Simplest  SaturateOnIntegerOverflow=off
  Data Type Conversion8 : DataTypeConversion  OutDataTypeStr=fixdt(1,24,20)  SaturateOnIntegerOverflow=off  RndMeth=Floor
  Delay1 : Delay  DelayLength=36
  Delay2 : Delay  DelayLength=21
  Delay22 : Delay  DelayLength=3
  Delay3 : Delay  DelayLength=66
  Delay4 : Delay  DelayLength=3
  Delay6 : Delay
  Delay_compensation : Subsystem  TreatAsAtomicUnit=on
  Delay_compensation_phase_currents : Scope  NumInputPorts=4
  Divide{,1..7} (8 alike) : Product  Inputs=*/  RndMeth=Zero  SaturateOnIntegerOverflow=on
  Index : Scope
  J : Scope
  J_min_Socpe : Scope  NumInputPorts=2
  Last_applied_phase_voltages : Scope
  Last_optimal_voltages : Scope  NumInputPorts=4
  Min_cost_funcion_vergleich : Scope  NumInputPorts=4
  Min_cost_function_and_vopt2 : Subsystem  TreatAsAtomicUnit=on
  Mux : Mux  Inputs=3
  Mux1 : Mux  Inputs=3
  Mux2 : Mux
  Mux3 : Mux
  Mux4 : Mux  Inputs=12
  Mux5 : Mux  Inputs=6
  Omega_el : Scope
  Phase_voltages_per_switching_state2 : Subsystem  TreatAsAtomicUnit=on
  Phase_voltages_per_switching_states : Scope
  Prediction_and_cost_function : Subsystem  TreatAsAtomicUnit=on
  Pulse Generator3 : DiscretePulseGenerator  PulseType=Time based  Period=1/f_c  PulseWidth=0.1
  Pulse Generator4 : DiscretePulseGenerator  Commented=on  PulseType=Time based  Period=1/100000  PulseWidth=5
  Rate Transition{1..23} (23 alike) : RateTransition  OutPortSampleTime=1.0000e-08
  Switching_states : Subsystem  TreatAsAtomicUnit=on
  Terminator{,1,6..7,9..10} (6 alike) : Terminator
  VSD_and_Park_transformed_phase_currents : Scope  NumInputPorts=4
  min_Index_AXI : Scope
  min_J_AXI : Scope
  phase_currents : Scope  NumInputPorts=8
  phase_currents1 : Scope  NumInputPorts=12
  phase_currents3 : Scope  NumInputPorts=2
  phase_currents_in_delay_compensation : Scope  NumInputPorts=2
  switching_state : Scope
  theta : Scope
  theta_test : Scope  NumInputPorts=2
  vsd_and_park_tra : Subsystem  TreatAsAtomicUnit=on
  HB1T1 : Outport
  HB1B1 : Outport  Port=2
  HB2T1 : Outport  Port=3
  HB2B1 : Outport  Port=4
  HB3T1 : Outport  Port=5
  HB3B1 : Outport  Port=6
  HB4T : Outport  Port=7
  HB4B : Outport  Port=8
  HB5T : Outport  Port=9
  HB5B : Outport  Port=10
  HB6T : Outport  Port=11
  HB6B : Outport  Port=12
  wires:
  Pulse Generator3/1 -> Data Type Conversion4/1
  vsd_and_park_tra/4(i_beta_axi) -> Terminator1/1
  vsd_and_park_tra/10(i_x_axi) -> [i_x_AXI]
  vsd_and_park_tra/16(i_0_minus_axi) -> Terminator7/1
  Constant1/1 -> Data Type Conversion10/1  "i_a1_IP_Core"
  vsd_and_park_tra/12(i_y_axi) -> [i_y_AXI]
  vsd_and_park_tra/14(i_0_plus_axi) -> Terminator6/1
  vsd_and_park_tra/8(i_q_axi) -> [i_q_AXI]
  vsd_and_park_tra/6(i_d_axi) -> [i_d_AXI]
  vsd_and_park_tra/2(i_alpha_axi) -> Terminator/1
  i_a1/1 -> Data Type Conversion7/1  "i_a1_IP_Core"
  i_c2/1 -> Data Type Conversion9/1  "i_c2_IP_Core"
  i_b2/1 -> Data Type Conversion6/1  "i_b2_IP_Core"
  i_a2/1 -> Data Type Conversion5/1  "i_a2_IP_Core"
  i_c1/1 -> Data Type Conversion3/1  "i_c1_IP_Core"
  i_b1/1 -> Data Type Conversion2/1  "i_b1_IP_Core"
  vsd_and_park_tra/1(i_alpha) -> Terminator9/1  "i_alpha"
  vsd_and_park_tra/3(i_beta) -> Terminator10/1  "i_beta"
  vsd_and_park_tra/13(i_0_plus) -> [i_0_plus]  "i_0_plus"
  vsd_and_park_tra/15(i_0_minus) -> [i_0_minus]  "i_0_minus"
  vsd_and_park_tra/18(i_a1_axi) -> [i_a1_AXI]
  vsd_and_park_tra/19(i_b1_axi) -> [i_b1_AXI]
  vsd_and_park_tra/20(i_c1_axi) -> [i_c1_AXI]
  vsd_and_park_tra/21(i_a2_axi) -> [i_a2_AXI]
  vsd_and_park_tra/22(i_b2_axi) -> [i_b2_AXI]
  vsd_and_park_tra/23(i_c2_axi) -> [i_c2_AXI]
  [i_a1_AXI] -> phase_currents1/1
  [i_b1_AXI] -> phase_currents1/2
  [i_c1_AXI] -> phase_currents1/3
  [i_a2_AXI] -> phase_currents1/4
  [i_b2_AXI] -> phase_currents1/5
  [i_c2_AXI] -> phase_currents1/6
  [i_d_AXI] -> VSD_and_Park_transformed_phase_currents/1
  [i_q_AXI] -> VSD_and_Park_transformed_phase_currents/2
  [i_y_AXI] -> VSD_and_Park_transformed_phase_currents/4
  [i_x_AXI] -> VSD_and_Park_transformed_phase_currents/3
  Divide1/1 -> Delay_compensation/7(SampleTime_div_Lq_AXI)
  Divide/1 -> Delay_compensation/6(SampleTime_div_Ld_AXI)
  Delay_compensation/2(iq_k_1) -> [iq_k_1]
  Divide2/1 -> Delay_compensation/8(SampleTime_div_Lx_AXI)
  Delay_compensation/1(id_k_1) -> [id_k_1]
  Delay_compensation/4(iy_k_1) -> [iy_k_1]
  Delay_compensation/3(ix_k_1) -> [ix_k_1]
  Divide3/1 -> Delay_compensation/9(SampleTime_div_Ly_AXI)
  psiPM/1 -> Rate Transition9/1  "i_d"
  Lq/1 -> Rate Transition10/1  "i_a1_IP_Core"
  Ld/1 -> Rate Transition11/1  "i_a1_IP_Core"
  Rs/1 -> Rate Transition12/1  "i_a1_IP_Core"
  Lx/1 -> Rate Transition14/1  "i_a1_IP_Core"
  Ly/1 -> Rate Transition15/1  "i_a1_IP_Core"
  pole_pairs/1 -> Rate Transition16/1  "i_a1_IP_Core"
  Constant/1 -> ?  "i_d"
  [valid_in_ADC] -> Delay_compensation/13(valid_in_ADC)
  vsd_and_park_tra/5(i_d) -> [i_d_measured]  "i_d"
  vsd_and_park_tra/7(i_q) -> [i_q_measured]  "i_q"
  vsd_and_park_tra/9(i_x) -> [i_x_measured]  "i_x"
  vsd_and_park_tra/11(i_y) -> [i_y_measured]  "i_y"
  Delay_compensation/6(id_k_1_AXI) -> [id_k_1_AXI]
  Delay_compensation/7(iq_k_1_AXI) -> [iq_k_1_AXI]
  Delay_compensation/8(ix_k_1_AXI) -> [ix_k_1_AXI]
  Delay_compensation/9(iy_k_1_AXI) -> [iy_k_1_AXI]
  [id_k_1_AXI] -> Delay_compensation_phase_currents/1
  [iq_k_1_AXI] -> Delay_compensation_phase_currents/2
  [ix_k_1_AXI] -> Delay_compensation_phase_currents/3
  [iy_k_1_AXI] -> Delay_compensation_phase_currents/4
  [theta_el] -> Phase_voltages_per_switching_state2/1(theta_el)
  [theta_el_offset_AXI] -> Phase_voltages_per_switching_state2/2(theta_el_offset_AXI)
  u_dc_link/1 -> Rate Transition22/1  "i_a1_IP_Core"
  [done_switching_states] -> Phase_voltages_per_switching_state2/5(valid_in_delay_compensation)
  [valid_in_ADC] -> Phase_voltages_per_switching_state2/7(valid_in_ADC)
  Phase_voltages_per_switching_state2/2(phase_voltages_per_switching_state) -> [phase_voltages_per_switching_states]
  [phase_voltages_per_switching_states] -> Phase_voltages_per_switching_states/1
  Divide6/1 -> Prediction_and_cost_function/5(SampleTime_div_Lx_AXI)
  [psiPM] -> Prediction_and_cost_function/14(psiPM_AXI)
  Divide7/1 -> Prediction_and_cost_function/6(SampleTime_div_Ly_AXI)
  [Ld] -> Divide4/2, Prediction_and_cost_function/2(Ld_AXI)
  [omega_m] -> Prediction_and_cost_function/12(omega_m_measured)
  [SampleTime] -> Divide5/1, Divide7/1, Divide6/1, Divide4/1
  [Lq] -> Divide5/2, Prediction_and_cost_function/1(Lq_AXI)
  Divide4/1 -> Prediction_and_cost_function/3(SampleTime_div_Ld_AXI)
  [Rs] -> Prediction_and_cost_function/11(Rs_AXI)
  [Ly] -> Divide7/2
  [Lx] -> Divide6/2
  Prediction_and_cost_function/2(Index) -> [Index]
  Divide5/1 -> Prediction_and_cost_function/4(SampleTime_div_Lq_AXI)
  [pole_pairs] -> Prediction_and_cost_function/13(pole_pairs_AXI)
  Prediction_and_cost_function/3(J) -> [J]
  [J] -> J/1
  [Index] -> Index/1
  [id_k_1] -> Prediction_and_cost_function/7(id_k_1)
  [iq_k_1] -> Prediction_and_cost_function/8(iq_k_1)
  [ix_k_1] -> Prediction_and_cost_function/9(ix_k_1)
  [iy_k_1] -> Prediction_and_cost_function/10(iy_k_1)
  id_ref/1 -> Rate Transition18/1  "i_a1_IP_Core"
  iq_ref/1 -> Rate Transition19/1  "i_a1_IP_Core"
  ix_ref/1 -> Rate Transition20/1  "i_a1_IP_Core"
  iy_ref/1 -> Rate Transition21/1  "i_a1_IP_Core"
  [valid_in_phase_voltages] -> Prediction_and_cost_function/19(valid_in)
  [done_VSD_and_Park] -> Prediction_and_cost_function/20(Reset)
  [valid_in_ADC] -> Prediction_and_cost_function/21(valid_in_ADC)
  [phase_voltages_per_switching_states] -> Prediction_and_cost_function/22(dqxy_phase_voltage_per_switching_state)
  Min_cost_function_and_vopt2/4(Index_AXI) -> [min_Index_AXI]
  Min_cost_function_and_vopt2/2(Index) -> [min_Index]
  Min_cost_function_and_vopt2/3(voltages) -> [last_applied_optimal_voltages]
  [Index] -> Min_cost_function_and_vopt2/1(Index_in)
  [Index] -> Phase_voltages_per_switching_state2/4(Index)
  [valid_in_prediction_and_cost_function] -> Min_cost_function_and_vopt2/2(valid_in)
  [J] -> Min_cost_function_and_vopt2/3(J_in)
  [phase_voltages_per_switching_states] -> Min_cost_function_and_vopt2/4(phase_voltages_per_switching_state_in)
  [min_J_AXI] -> min_J_AXI/1
  [min_Index_AXI] -> min_Index_AXI/1
  [last_applied_optimal_voltages] -> Last_applied_phase_voltages/1
  [last_applied_optimal_voltages] -> Delay_compensation/10(last_applied_optimal_voltages_in)
  [valid_in_done_min_cost_function] -> Phase_voltages_per_switching_state2/6(valid_in_min_cost_function-and_vopt)
  [min_Index] -> Switching_states/1(I)
  [valid_in_ADC] -> Ablauf/1  "valid_in_ADC"
  [done_VSD_and_Park] -> Ablauf/2  "done_VSD_and_Park"
  [valid_in_delay_compensation] -> Ablauf/3  "done_delay_compensation"
  [valid_in_phase_voltages] -> Ablauf/4  "done_phase_voltages"
  [valid_in_prediction_and_cost_function] -> Ablauf/5  "done_prediction_and_cost_function"
  [valid_in_done_min_cost_function] -> Ablauf/6  "done_min_cost_function"
  [done_switching_states] -> Ablauf/7  "done_switching_states"
  Switching_states/13(done) -> [done_switching_states]
  [id_k_1_AXI] -> phase_currents/1  "id_k_1"
  [iq_k_1_AXI] -> phase_currents/2  "iq_k_1"
  [ix_k_1_AXI] -> phase_currents/3  "ix_k_1"
  [iy_k_1_AXI] -> phase_currents/4  "iy_k_1"
  [i_d_AXI] -> phase_currents/5  "id"
  [i_q_AXI] -> phase_currents/6  "iq"
  [i_x_AXI] -> phase_currents/7  "ix"
  [i_y_AXI] -> phase_currents/8  "iy"
  Data Type Conversion4/1 -> Rate Transition8/1  "i_a1_IP_Core"
  SampleTime/1 -> Rate Transition13/1  "i_a1_IP_Core"
  [i_a1] -> phase_currents1/7
  [i_b1] -> phase_currents1/8
  [i_c1] -> phase_currents1/9
  [i_a2] -> phase_currents1/10
  [i_b2] -> phase_currents1/11
  [i_c2] -> phase_currents1/12
  vsd_and_park_tra/24(theta_test) -> [theta_test_vsd]
  [theta_test_vsd] -> theta_test/1  "VSD"
  Phase_voltages_per_switching_state2/3(theta_test) -> theta/1, [theta_test_phase_voltages]
  [theta_test_phase_voltages] -> theta_test/2  "phase_voltages"
  theta_el/1 -> Data Type Conversion11/1  "i_a1_IP_Core"
  [id_k_1] -> Mux2/1
  [iq_k_1] -> Mux2/2
  [ix_k_1] -> Mux2/3
  [iy_k_1] -> Mux2/4
  Mux2/1 -> phase_currents3/2
  [last_applied_optimal_voltage_d] -> Last_optimal_voltages/1
  Delay_compensation/10(last_applied_optimal_voltage_d) -> [last_applied_optimal_voltage_d]
  Delay_compensation/11(last_applied_optimal_voltage_q) -> [last_applied_optimal_voltage_q]
  Delay_compensation/12(last_applied_optimal_voltage_x) -> [last_applied_optimal_voltage_x]
  Delay_compensation/13(last_applied_optimal_voltage_y) -> [last_applied_optimal_voltage_y]
  [last_applied_optimal_voltage_q] -> Last_optimal_voltages/2
  [last_applied_optimal_voltage_x] -> Last_optimal_voltages/3
  [last_applied_optimal_voltage_y] -> Last_optimal_voltages/4
  Delay_compensation/14(measured_currents_delay_compensation) -> [measured_currents_delay_compensation]
  Prediction_and_cost_function/7(iy_k_1_Prediction) -> Mux3/4
  Prediction_and_cost_function/6(ix_k_1_Prediction) -> Mux3/3
  Prediction_and_cost_function/4(id_k_1_Prediction) -> Mux3/1
  Prediction_and_cost_function/5(iq_k_1_Prediction) -> Mux3/2
  Mux3/1 -> [i_dqxy_k_1_Prediction]
  [i_dqxy_k_1_Prediction] -> phase_currents_in_delay_compensation/2
  [measured_currents_delay_compensation] -> phase_currents_in_delay_compensation/1
  vsd_and_park_tra/17(done) -> [done_VSD_and_Park]
  [done_VSD_and_Park] -> Delay_compensation/14(valid_in)
  [i_d_measured] -> Data Type Conversion19/1
  [i_x_measured] -> Data Type Conversion21/1
  [i_y_measured] -> Data Type Conversion22/1
  Rate Transition23/1 -> [i_a1], Mux/1  "i_a1_IP_Core"
  Rate Transition1/1 -> Mux/2, [i_b1]  "i_a1_IP_Core"
  Rate Transition2/1 -> [i_c1], Mux/3  "i_a1_IP_Core"
  Rate Transition3/1 -> Mux1/1, [i_a2]  "i_a1_IP_Core"
  Rate Transition4/1 -> [i_b2], Mux1/2  "i_a1_IP_Core"
  Rate Transition5/1 -> [i_c2], Mux1/3  "i_a1_IP_Core"
  Rate Transition6/1 -> vsd_and_park_tra/3(theta_el), [theta_el]  "i_a1_IP_Core"
  Rate Transition7/1 -> vsd_and_park_tra/4(theta_el_offset_), [theta_el_offset_AXI]  "i_a1_IP_Core"
  Rate Transition8/1 -> [valid_in_ADC], vsd_and_park_tra/5(curent_valid_in)  "i_a1_IP_Core"
  Rate Transition9/1 -> [psiPM], Delay_compensation/2(psiPM_AXI)  "i_a1_IP_Core"
  Rate Transition10/1 -> [Lq], Delay_compensation/3(Lq_AXI), Divide1/2  "i_a1_IP_Core"
  Rate Transition11/1 -> [Ld], Delay_compensation/4(Ld_AXI), Divide/2  "i_a1_IP_Core"
  Rate Transition12/1 -> [Rs], Delay_compensation/5(Rs_AXI)  "i_a1_IP_Core"
  Rate Transition13/1 -> Divide/1, Divide1/1, Divide3/1, Divide2/1, [SampleTime]  "i_a1_IP_Core"
  Rate Transition14/1 -> [Lx], Divide2/2  "i_a1_IP_Core"
  Rate Transition15/1 -> [Ly], Divide3/2  "i_a1_IP_Core"
  Rate Transition16/1 -> [pole_pairs], Delay_compensation/11(pole_pairs_AXI)  "i_a1_IP_Core"
  Rate Transition17/1 -> [omega_m], Delay_compensation/12(omega_m_measured)  "i_a1_IP_Core"
  Rate Transition18/1 -> Prediction_and_cost_function/15(id_ref_AXI)  "i_a1_IP_Core"
  Rate Transition19/1 -> Prediction_and_cost_function/16(iq_ref_AXI)  "i_a1_IP_Core"
  Rate Transition20/1 -> Prediction_and_cost_function/17(ix_ref_AXI)  "i_a1_IP_Core"
  Rate Transition21/1 -> Prediction_and_cost_function/18(iy_ref_AXI)  "i_a1_IP_Core"
  Rate Transition22/1 -> Phase_voltages_per_switching_state2/3(u_dc_link_voltage_AXI)  "i_a1_IP_Core"
  [min_J_AXI] -> J_min_Socpe/2
  Switching_states/1(HB1T) -> HB1T1/1, Mux4/1
  Switching_states/2(HB1B) -> HB1B1/1, Mux4/2
  Switching_states/3(HB2T) -> HB2T1/1, Mux4/3
  Switching_states/4(HB2B) -> HB2B1/1, Mux4/4
  Switching_states/5(HB3T) -> HB3T1/1, Mux4/5
  Switching_states/6(HB3B) -> HB3B1/1, Mux4/6
  Switching_states/7(HB4T) -> HB4T/1, Mux4/7
  Switching_states/8(HB4B) -> HB4B/1, Mux4/8
  Switching_states/9(HB5T) -> HB5T/1, Mux4/9
  Switching_states/10(HB5B) -> HB5B/1, Mux4/10
  Switching_states/11(HB6T) -> Mux4/11, HB6T/1
  Switching_states/12(HB6B) -> Mux4/12, HB6B/1
  Mux4/1 -> [Schaltstellung]
  [Schaltstellung] -> switching_state/1
  Delay_compensation/15(omega_el) -> [omega_el]
  [omega_el] -> Omega_el/1
  [min_Index] -> Min_cost_funcion_vergleich/1  "min_Index"
  [min_J_AXI] -> Min_cost_funcion_vergleich/2  "min_J"
  [j_min_test] -> Min_cost_funcion_vergleich/3  "min_J_test"
  [last_applied_optimal_voltages] -> Min_cost_funcion_vergleich/4  "voltages"
  [valid_in_delay_compensation] -> Switching_states/2(valid_in)
  [done_switching_states] -> ?
  Data Type Conversion7/1 -> Rate Transition23/1  "fc"
  Data Type Conversion2/1 -> Rate Transition1/1  "fc"
  Data Type Conversion3/1 -> Rate Transition2/1  "fc"
  Data Type Conversion5/1 -> Rate Transition3/1  "fc"
  Data Type Conversion6/1 -> Rate Transition4/1  "fc"
  Data Type Conversion9/1 -> Rate Transition5/1  "fc"
  Data Type Conversion10/1 -> Rate Transition7/1
  Prediction_and_cost_function/1(done) -> [valid_in_prediction_and_cost_function]
  Min_cost_function_and_vopt2/1(done) -> [valid_in_done_min_cost_function]
  Phase_voltages_per_switching_state2/1(done) -> [valid_in_phase_voltages]
  Delay_compensation/5(done) -> [valid_in_delay_compensation]
  Data Type Conversion11/1 -> Rate Transition6/1
  [i_q_measured] -> Data Type Conversion20/1  "fc"
  Mux/1 -> vsd_and_park_tra/1(abc_1)
  Mux1/1 -> vsd_and_park_tra/2(abc_2)
  [i_0_plus] -> Data Type Conversion23/1
  [i_0_minus] -> Data Type Conversion24/1
  Data Type Conversion19/1 -> Mux5/1  "fc"
  Data Type Conversion20/1 -> Mux5/2  "fc"
  Data Type Conversion21/1 -> Mux5/3  "fc"
  Data Type Conversion22/1 -> Mux5/4  "fc"
  Data Type Conversion23/1 -> Mux5/5  "fc"
  Data Type Conversion24/1 -> Mux5/6  "fc"
  Mux5/1 -> Delay_compensation/1(dq_measured_currents)
  omega_m/1 -> Rate Transition17/1  "i_d"

== system FCS_MPC_6ph_CIL_FCS_reduced/Power_Source ==
  Controlled Voltage Source : fl_lib/Electrical/Electrical Sources/Controlled Voltage Source
      settings: SourceProductBaseCode=PW,SS,VE
  + : PMIOPort  Side=Right
  - : PMIOPort  Port=2  Side=Right
  ref_voltage : PMIOPort  Port=3  Side=Left
  connections:
  Controlled Voltage Source/LConn1 -- +/RConn1
  Controlled Voltage Source/RConn2 -- -/RConn1
  Controlled Voltage Source/RConn1 -- ref_voltage/RConn1
